simulink model "controllerVodorod"  (R2018b)
settings: Solver=VariableStepAuto  StartTime=0.0  StopTime=10.0  RelTol=1e-3
settings Model: Creator=K2  LastModifiedBy=K2

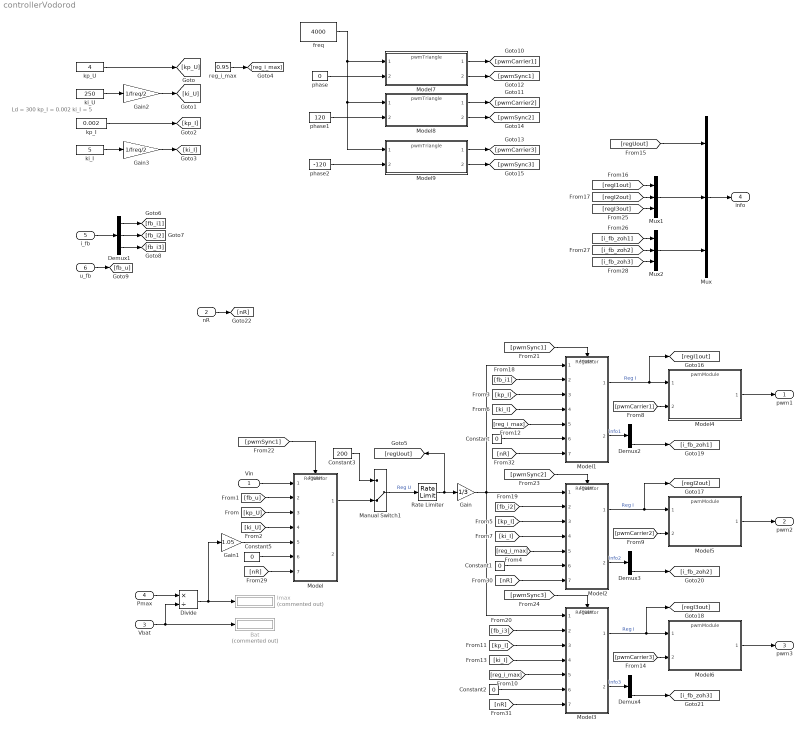
== system controllerVodorod ==
  note: Ld = 300
      | kp_I = 0.002
      | ki_I = 5
  Vin : Inport
  nR : Inport  Port=2
  Vbat : Inport  Port=3
  Pmax : Inport  Port=4
  i_fb : Inport  Port=5
  u_fb : Inport  Port=6
  Bat : Display  Commented=on
      settings: Format=bank
  Constant{,1..2,5} (4 alike) : Constant  Value=0
  Constant3 : Constant  Value=200
  Demux1 : Demux  Outputs=3
  Demux2 : Demux
  Demux3 : Demux
  Demux4 : Demux
  Divide : Product  Inputs=*/
  Gain : Gain  Gain=1/3
  Gain1 : Gain  Gain=1.05
  Gain2 : Gain  Gain=1/freq/2
  Gain3 : Gain  Gain=1/freq/2
  Imax : Display  Commented=on
      settings: Format=bank
  Manual Switch1 : ManualSwitch  CurrentSetting=0
  Model{,1..3} (4 alike) : ModelReference  ModelNameDialog=Regulator.slx  SimulationMode=Normal  ModelReferenceVersion=1.46  TriggerPortName=Trigger  TriggerPortTriggerType=either
  Model4 : ModelReference  ModelNameDialog=pwmModule.slx  SimulationMode=Normal  ModelReferenceVersion=1.3
  Model5 : ModelReference  ModelNameDialog=pwmModule.slx  SimulationMode=Normal  ModelReferenceVersion=1.3
  Model6 : ModelReference  ModelNameDialog=pwmModule.slx  SimulationMode=Normal  ModelReferenceVersion=1.3
  Model7 : ModelReference  ModelNameDialog=pwmTriangle.slx  SimulationMode=Normal  ModelReferenceVersion=1.5
  Model8 : ModelReference  ModelNameDialog=pwmTriangle.slx  SimulationMode=Normal  ModelReferenceVersion=1.5
  Model9 : ModelReference  ModelNameDialog=pwmTriangle.slx  SimulationMode=Normal  ModelReferenceVersion=1.5
  Mux : Mux  Inputs=3
  Mux1 : Mux  Inputs=3
  Mux2 : Mux  Inputs=3
  Rate Limiter : RateLimiter  RisingSlewLimit=1000  FallingSlewLimit=-100000  SampleTimeMode=inherited
  freq : Constant  Value=4000
  ki_I : Constant  Value=5
  ki_U : Constant  Value=250
  kp_I : Constant  Value=0.002
  kp_U : Constant  Value=4
  phase : Constant  Value=0
  phase1 : Constant  Value=120
  phase2 : Constant  Value=-120
  reg_i_max : Constant  Value=0.95
  pwm1 : Outport
  pwm2 : Outport  Port=2
  pwm3 : Outport  Port=3
  info : Outport  Port=4  OutDataTypeStr=double
  wires:
  ki_U/1 -> Gain2/1
  [pwmCarrier2] -> Model5/2
  [pwmCarrier3] -> Model6/2
  [pwmSync2] -> Model2/Trigger
  [pwmSync1] -> Model/Trigger
  [pwmSync3] -> Model3/Trigger
  [reg_i_max] -> Model1/5
  Constant3/1 -> Manual Switch1/1
  [kp_U] -> Model/3
  [reg_i_max] -> Model3/5
  Divide/1 -> Gain1/1, Imax/1
  kp_I/1 -> [kp_I]
  Gain1/1 -> Model/5
  [pwmSync1] -> Model1/Trigger
  [pwmCarrier1] -> Model4/2
  Model8/1 -> [pwmCarrier2]
  [reg_i_max] -> Model2/5
  Demux1/3 -> [fb_i3]
  Gain/1 -> Model1/1, Model3/1, Model2/1
  [fb_i1] -> Model1/2
  Gain2/1 -> [ki_U]
  [ki_U] -> Model/4
  phase/1 -> Model7/2
  Demux1/1 -> [fb_i1]
  [fb_u] -> Model/2
  Model9/2 -> [pwmSync3]
  i_fb/1 -> Demux1/1
  [fb_i2] -> Model2/2
  Model/1 -> Manual Switch1/2
  Model8/2 -> [pwmSync2]
  [kp_I] -> Model3/3
  [ki_I] -> Model3/4
  Gain3/1 -> [ki_I]
  phase2/1 -> Model9/2
  Constant1/1 -> Model2/6
  Model9/1 -> [pwmCarrier3]
  [ki_I] -> Model1/4
  Demux1/2 -> [fb_i2]
  [fb_i3] -> Model3/2
  Model7/1 -> [pwmCarrier1]
  Pmax/1 -> Divide/1
  Constant/1 -> Model1/6
  [ki_I] -> Model2/4
  [kp_I] -> Model1/3
  Model4/1 -> pwm1/1
  Model6/1 -> pwm3/1
  reg_i_max/1 -> [reg_i_max]
  phase1/1 -> Model8/2
  Constant5/1 -> Model/6
  Model5/1 -> pwm2/1
  ki_I/1 -> Gain3/1
  Model7/2 -> [pwmSync1]
  Vbat/1 -> Divide/2, Bat/1
  Model1/1 -> [regI1out], Model4/1  "Reg I"
  freq/1 -> Model8/1, Model9/1, Model7/1
  Constant2/1 -> Model3/6
  [kp_I] -> Model2/3
  u_fb/1 -> [fb_u]
  Vin/1 -> Model/1
  Manual Switch1/1 -> Rate Limiter/1  "Reg U"
  Rate Limiter/1 -> Gain/1, [regUout]
  kp_U/1 -> [kp_U]
  Mux/1 -> info/1
  [regUout] -> Mux/1
  [regI1out] -> Mux1/1
  Model2/1 -> [regI2out], Model5/1  "Reg I"
  Model3/1 -> [regI3out], Model6/1  "Reg I"
  [regI2out] -> Mux1/2
  [regI3out] -> Mux1/3
  Mux1/1 -> Mux/2
  [i_fb_zoh2] -> Mux2/2
  [i_fb_zoh1] -> Mux2/1
  [i_fb_zoh3] -> Mux2/3
  Model1/2 -> Demux2/1  "info1"
  Model2/2 -> Demux3/1  "info2"
  Model3/2 -> Demux4/1  "info3"
  Demux2/4 -> [i_fb_zoh1]
  Demux3/4 -> [i_fb_zoh2]
  Demux4/4 -> [i_fb_zoh3]
  Mux2/1 -> Mux/3
  nR/1 -> [nR]
  [nR] -> Model/7
  [nR] -> Model2/7
  [nR] -> Model3/7
  [nR] -> Model1/7
